simulink model "cascaded_multilevel (1)"  (R2015a)
settings: Solver=ode45  StartTime=0.0  StopTime=0.04  RelTol=1e-3
libraries: powerlib x15, simulink x4
settings Model: Creator=User  LastModifiedBy=User

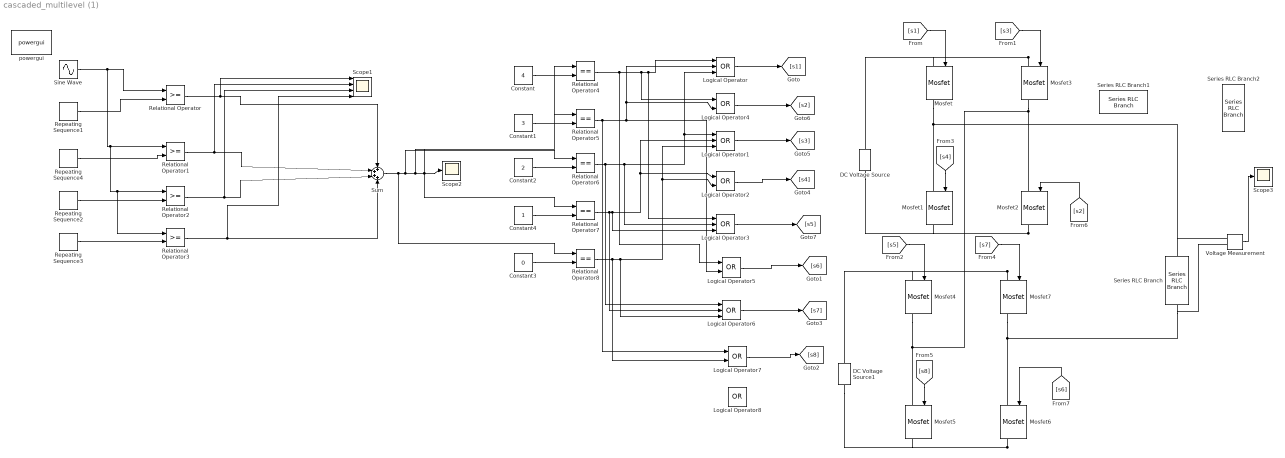
== system cascaded_multilevel (1) ==
  Constant : Constant  Value=4
  Constant1 : Constant  Value=3
  Constant2 : Constant  Value=2
  Constant3 : Constant  Value=0
  Constant4 : Constant
  DC Voltage Source : powerlib/Electrical Sources/DC Voltage Source  Amplitude=400  Measurements=None
  DC Voltage Source1 : powerlib/Electrical Sources/DC Voltage Source  Amplitude=400  Measurements=None
  Logical Operator{,1,3,6,8} (5 alike) : Logic  Operator=OR  Inputs=3  AllPortsSameDT=off  OutDataTypeStr=boolean
  Logical Operator{2,4..5,7} (4 alike) : Logic  Operator=OR  AllPortsSameDT=off  OutDataTypeStr=boolean
  Mosfet{,1..7} (8 alike) : powerlib/Power Electronics/Mosfet  Ron=0.1  Lon=0  Rd=0.01  Vfd=0  IC=0  Rs=1e5  Cs=inf  Measurements=on
  Relational Operator{,1..3} (4 alike) : RelationalOperator  OutDataTypeStr=boolean
  Relational Operator{4..8} (5 alike) : RelationalOperator  Operator===  OutDataTypeStr=boolean
  Repeating Sequence1 : simulink/Sources/Repeating Sequence  rep_seq_t=[0 1 2]*[1/400]  rep_seq_y=[1 2 1]
  Repeating Sequence2 : simulink/Sources/Repeating Sequence  rep_seq_t=[0 1 2]*[1/400]  rep_seq_y=[-1 0 -1]
  Repeating Sequence3 : simulink/Sources/Repeating Sequence  rep_seq_t=[0 1 2]*[1/400]  rep_seq_y=[-2 -1 -2]
  Repeating Sequence4 : simulink/Sources/Repeating Sequence  rep_seq_t=[0 1 2]*[1/400]  rep_seq_y=[0 1 0]
  Scope1 : Scope  NumInputPorts=4
      settings: YMin=-5~-5~-5~-5  YMax=5~5~5~5
  Scope2 : Scope
      settings: SaveName=ScopeData2
  Scope3 : Scope
      settings: SaveName=tamzid
  Series RLC Branch : powerlib/Elements/Series RLC Branch  LConnTagsString=__new0  RConnTagsString=__new0  BranchType=R  Resistance=200  Inductance=1e-3  SetiL0=off  InitialCurrent=0  Capacitance=1e-6  Setx0=off  InitialVoltage=0  Measurements=None
  Series RLC Branch1 : powerlib/Elements/Series RLC Branch  LConnTagsString=__new0  RConnTagsString=__new0  BranchType=L  Resistance=5  Inductance=1e-3  SetiL0=off  InitialCurrent=0  Capacitance=1e-6  Setx0=off  InitialVoltage=0  Measurements=None
  Series RLC Branch2 : powerlib/Elements/Series RLC Branch  LConnTagsString=__new0  RConnTagsString=__new0  BranchType=C  Resistance=5  Inductance=1e-3  SetiL0=off  InitialCurrent=0  Capacitance=1e-6  Setx0=off  InitialVoltage=0  Measurements=None
  Sine Wave : Sin  Amplitude=2  Frequency=2*pi*50  SampleTime=0
  Sum : Sum  Inputs=4
  Voltage Measurement : powerlib/Measurements/Voltage Measurement  PhasorSimulation=off  OutputType=Complex  PSBequivalent=0
  powergui : powerlib/powergui  Priority=1  SimulationMode=Continuous  SolverType=Tustin/Backward Euler (TBE)  SampleTime=50e-6  frequency=60  SPID=off  DisableSnubberDevices=off  DisableRonSwitches=off  DisableVfSwitches=off  SwTol=0  DisplayEquations=off  Interpol=off  methode=off  Ts=100  FunctionMessages=off  echomessages=off  HookPort=off  EnableUseOfTLC=off  x0status=blocks  frequencyindice=0  Pbase=100e6  ErrMax=1e-4  Iterations=50  UnitsV=kV  UnitsW=MW  buscounter=0  RestoreLinks=warning  ResistiveCurrentMeasurement=off  Frange=[0:2:500]  Ylog=off  Xlog=on  ShowGrid=off  save=off  variable=ZData  structure=tamzid  ZoomFFT=off  StartTime=0.0  cycles=2  DisplayStyle=1  fundamental=50  FreqAxis=off  MaxFrequency=1000  frequencyindicesteady=1  RmsSteady=1  display=off
  wires:
  Sine Wave/1 -> Relational Operator3/1, Relational Operator2/1, Relational Operator1/1, Relational Operator/1
  Repeating Sequence1/1 -> Relational Operator/2
  Repeating Sequence4/1 -> Relational Operator1/2
  Repeating Sequence2/1 -> Relational Operator2/2
  Repeating Sequence3/1 -> Relational Operator3/2
  Relational Operator/1 -> Scope1/1, Sum/1
  Relational Operator1/1 -> Scope1/2, Sum/2
  Relational Operator2/1 -> Scope1/3, Sum/3
  Relational Operator3/1 -> Scope1/4, Sum/4
  Sum/1 -> Relational Operator8/1, Relational Operator6/1, Relational Operator5/1, Relational Operator7/1, Relational Operator4/1, Scope2/1
  Constant/1 -> Relational Operator4/2
  Constant1/1 -> Relational Operator5/2
  Constant2/1 -> Relational Operator6/2
  Constant4/1 -> Relational Operator7/2
  Constant3/1 -> Relational Operator8/2
  Relational Operator4/1 -> Logical Operator5/1, Logical Operator4/1, Logical Operator3/1, Logical Operator/1
  Relational Operator5/1 -> Logical Operator7/1, Logical Operator5/2, Logical Operator4/2, Logical Operator/2
  Relational Operator6/1 -> Logical Operator6/1, Logical Operator3/2, Logical Operator1/1, Logical Operator/3
  Relational Operator7/1 -> Logical Operator6/2, Logical Operator3/3, Logical Operator2/1, Logical Operator1/2
  Relational Operator8/1 -> Logical Operator7/2, Logical Operator6/3, Logical Operator2/2, Logical Operator1/3
  Logical Operator/1 -> [s1]
  Logical Operator4/1 -> [s2]
  Logical Operator1/1 -> [s3]
  Logical Operator2/1 -> [s4]
  Logical Operator3/1 -> [s5]
  Logical Operator5/1 -> [s6]
  Logical Operator6/1 -> [s7]
  Logical Operator7/1 -> [s8]
  [s1] -> Mosfet/1
  [s3] -> Mosfet3/1
  [s4] -> Mosfet1/1
  [s5] -> Mosfet4/1
  [s7] -> Mosfet7/1
  [s8] -> Mosfet5/1
  [s2] -> Mosfet2/1
  [s6] -> Mosfet6/1
  Voltage Measurement/1 -> Scope3/1
  connections:
  Mosfet/RConn1 -- Voltage Measurement/LConn1 -- Series RLC Branch/LConn1 -- Mosfet1/LConn1
  Mosfet3/LConn1 -- DC Voltage Source/RConn1 -- Mosfet/LConn1
  Mosfet2/RConn1 -- DC Voltage Source/LConn1 -- Mosfet1/RConn1
  Mosfet7/LConn1 -- DC Voltage Source1/RConn1 -- Mosfet4/LConn1
  Mosfet6/RConn1 -- DC Voltage Source1/LConn1 -- Mosfet5/RConn1
  Mosfet3/RConn1 -- Mosfet5/LConn1 -- Mosfet4/RConn1 -- Mosfet2/LConn1
  Mosfet7/RConn1 -- Voltage Measurement/LConn2 -- Series RLC Branch/RConn1 -- Mosfet6/LConn1
